simulink model "state_estimator"  (R2019a)
settings: Solver=ode4  StartTime=0.0  StopTime=endtime  FixedStep=0.001  RelTol=1e-3
values from neighbouring files (symbols this model uses):
  bike_m = bike    [Untitled2.m]
settings Model: Creator=chris  LastModifiedBy=chris

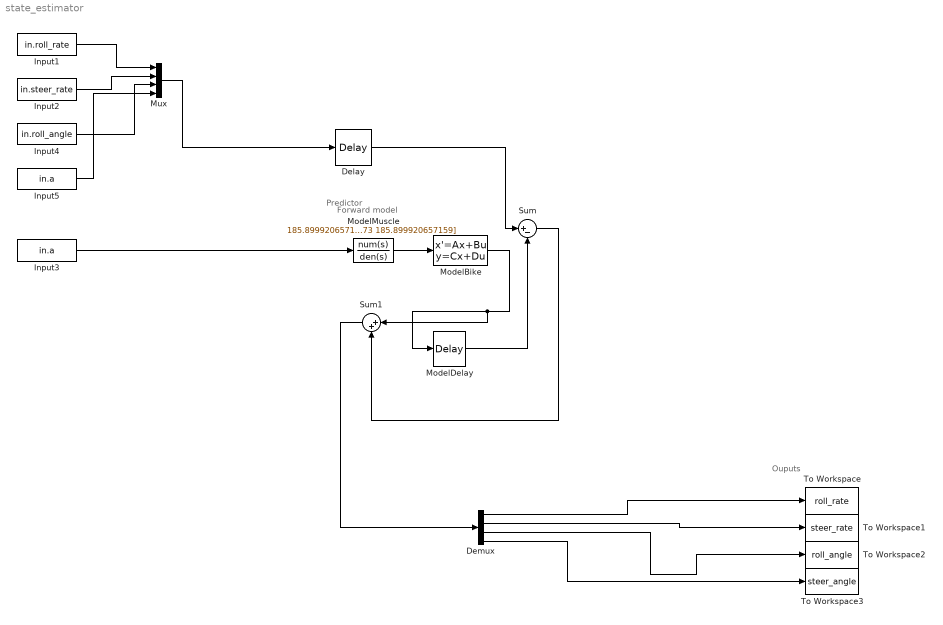
== system state_estimator ==
  note: Predictor
  note: Forward model
  note: Ouputs
  " ModelDelay " : TransportDelay  DelayTime=0.025
  Delay : TransportDelay  DelayTime=0.025
  Demux : Demux
  Input1 : FromWorkspace  VariableName=in.roll_rate  SampleTime=0
  Input2 : FromWorkspace  VariableName=in.steer_rate  SampleTime=0
  Input3 : FromWorkspace  VariableName=in.a  SampleTime=0
  Input4 : FromWorkspace  VariableName=in.roll_angle  SampleTime=0
  Input5 : FromWorkspace  VariableName=in.a  SampleTime=0
  "ModelBike " : StateSpace  A=bike_m.A  B=bike_m.B(:,2)  C=[1 0 0 0;0 1 0 0;0 0 1 0;0 0 0 1]  D=[0;0;0;0]  InitialCondition=0
  ModelMuscle : TransferFcn  Numerator=185.899920657159  Denominator=[1 19.2821119516073 185.899920657159]
  Mux : Mux
  Sum : Sum  Inputs=|+-
  Sum1 : Sum  Inputs=|++
  To Workspace : ToWorkspace  VariableName=roll_rate  SampleTime=-1
  To Workspace1 : ToWorkspace  VariableName=steer_rate  SampleTime=-1
  To Workspace2 : ToWorkspace  VariableName=roll_angle  SampleTime=-1
  To Workspace3 : ToWorkspace  VariableName=steer_angle  SampleTime=-1
  wires:
  Mux/1 -> Delay/1
  " ModelDelay "/1 -> Sum/2
  Sum1/1 -> Demux/1
  Delay/1 -> Sum/1
  "ModelBike "/1 -> " ModelDelay "/1, Sum1/1
  Sum/1 -> Sum1/2
  ModelMuscle/1 -> "ModelBike "/1
  Input3/1 -> ModelMuscle/1
  Input1/1 -> Mux/1
  Input2/1 -> Mux/2
  Input4/1 -> Mux/3
  Input5/1 -> Mux/4
  Demux/1 -> To Workspace/1
  Demux/2 -> To Workspace1/1
  Demux/4 -> To Workspace3/1
  Demux/3 -> To Workspace2/1
